simulink library "inp"  (R2021b)
settings: Solver=VariableStepAuto  StartTime=0.0  StopTime=10.0  RelTol=1e-3
undefined symbols (not defined in the file): C_TASK_5MS_S, FALSE, KINP_AcoreReadyToSlp_flg_ovrdflg, KINP_AcoreReadyToSlp_flg_ovrdval, KINP_AllowMovThd_OTA_enum_ovrdflg, KINP_AllowMovThd_OTA_enum_ovrdval, KINP_APSAngleTarget_Deg_ovrdflg, KINP_APSAngleTarget_Deg_ovrdval, KINP_APSDecReq_mps2_ovrdflg, KINP_APSDecReq_mps2_ovrdval, KINP_APSDecReqA_flg_ovrdflg, KINP_APSDecReqA_flg_ovrdval, KINP_APSDFLL_cm_ovrdflg, KINP_APSDFLL_cm_ovrdval, KINP_APSDFLR_cm_ovrdflg, KINP_APSDFLR_cm_ovrdval, KINP_APSDRLL_cm_ovrdflg, KINP_APSDRLL_cm_ovrdval, KINP_APSDRLR_cm_ovrdflg, KINP_APSDRLR_cm_ovrdval, KINP_APSExitCondition_enum_ovrdflg, KINP_APSExitCondition_enum_ovrdval, KINP_APSHWVer_enum_ovrdflg, KINP_APSHWVer_enum_ovrdval, KINP_APSProgressPCT_pct_ovrdflg, KINP_APSProgressPCT_pct_ovrdval, KINP_APSPwrReq_enum_ovrdflg, KINP_APSPwrReq_enum_ovrdval, KINP_APSReq_enum_ovrdflg, KINP_APSReq_enum_ovrdval, KINP_APSRQDisplay_enum_ovrdflg, KINP_APSRQDisplay_enum_ovrdval, KINP_APSRqEPASCtrl_flg_ovrdflg, KINP_APSRqEPASCtrl_flg_ovrdval, KINP_APSShiftPosnReq_enum_ovrdval, KINP_APSShiftPosnReq_enum_ovrflg, KINP_APSSpeedCMD_kph_ovrdval, KINP_APSSpeedCMD_kph_ovrflg, KINP_APSStaSystem_enum_ovrdflg, KINP_APSStaSystem_enum_ovrdval, KINP_APSSWVer_enum_ovrdflg, KINP_APSSWVer_enum_ovrdval, KINP_APSVMCReqA_flg_ovrdval, KINP_APSVMCReqA_flg_ovrflg, KINP_APSVRqEPASCtrl_flg_ovrdflg, KINP_APSVRqEPASCtrl_flg_ovrdval, KINP_AuxBattVolmV_mV_ovrdflg, KINP_AuxBattVolmV_mV_ovrdval, KINP_BTConnectSta_enum_ovrdflg, KINP_BTConnectSta_enum_ovrdval, KINP_CAASSta_enum_ovrdflg, KINP_CAASSta_enum_ovrdval, KINP_CAASVMCReqA_flg_ovrdval, KINP_CAASVMCReqA_flg_ovrflg, KINP_CAN1BusOff_flg_ovrdflg, KINP_CAN1BusOff_flg_ovrdval, KINP_CAN2BusOff_flg_ovrdflg, KINP_CAN2BusOff_flg_ovrdval, KINP_CAN3BusOff_flg_ovrdflg, KINP_CAN3BusOff_flg_ovrdval ... (+222)
libraries: FVT_lib x1035, hcu_lib x1
(part 25 of 33)

== system inp/INP/CAN3/SignalCheck/MCU_N_R2 ==
  BHAL_outputs : Inport
  inp_CanValid_bus : Inport  Port=2
  RrCoolanttempReqNidec : FVT_lib/inp/can_signal_template  SystemSampleTime=-1  VariantActivationTime=update diagram  Latency=0  AutoFrameSizeCalculation=off
      link override defval: Value=KINP_RrCoolanttempReqNidec_cnt_defval
      link override ovrdflg: Value=KINP_RrCoolanttempReqNidec_cnt_ovrdflg
      link override ovrdval: Value=KINP_RrCoolanttempReqNidec_cnt_ovrdval
  RrEOPSpdSetNidec : FVT_lib/inp/can_signal_template  SystemSampleTime=-1  VariantActivationTime=update diagram  Latency=0  AutoFrameSizeCalculation=off
      link override defval: Value=KINP_RrEOPSpdSetNidec_rpm_defval
      link override ovrdflg: Value=KINP_RrEOPSpdSetNidec_rpm_ovrdflg
      link override ovrdval: Value=KINP_RrEOPSpdSetNidec_rpm_ovrdval
  RrFailcode1Nidec : FVT_lib/inp/can_signal_template  SystemSampleTime=-1  VariantActivationTime=update diagram  Latency=0  AutoFrameSizeCalculation=off
      link override defval: Value=KINP_RrFailcode1Nidec_enum_defval
      link override ovrdflg: Value=KINP_RrFailcode1Nidec_enum_ovrdflg
      link override ovrdval: Value=KINP_RrFailcode1Nidec_enum_ovrdval
  RrFailcode2Nidec : FVT_lib/inp/can_signal_template  SystemSampleTime=-1  VariantActivationTime=update diagram  Latency=0  AutoFrameSizeCalculation=off
      link override defval: Value=KINP_RrFailcode2Nidec_enum_defval
      link override ovrdflg: Value=KINP_RrFailcode2Nidec_enum_ovrdflg
      link override ovrdval: Value=KINP_RrFailcode2Nidec_enum_ovrdval
  RrFailcodehistory1Nidec : FVT_lib/inp/can_signal_template  SystemSampleTime=-1  VariantActivationTime=update diagram  Latency=0  AutoFrameSizeCalculation=off
      link override defval: Value=KINP_RrFailcodehistory1Nidec_enum_defval
      link override ovrdflg: Value=KINP_RrFailcodehistory1Nidec_enum_ovrdflg
      link override ovrdval: Value=KINP_RrFailcodehistory1Nidec_enum_ovrdval
  RrFailcodehistory2Nidec : FVT_lib/inp/can_signal_template  SystemSampleTime=-1  VariantActivationTime=update diagram  Latency=0  AutoFrameSizeCalculation=off
      link override defval: Value=KINP_RrFailcodehistory2Nidec_enum_defval
      link override ovrdflg: Value=KINP_RrFailcodehistory2Nidec_enum_ovrdflg
      link override ovrdval: Value=KINP_RrFailcodehistory2Nidec_enum_ovrdval
  RrLLCTempNidec : FVT_lib/inp/can_signal_template  SystemSampleTime=-1  VariantActivationTime=update diagram  Latency=0  AutoFrameSizeCalculation=off
      link override defval: Value=KINP_RrLLCTempNidec_C_defval
      link override ovrdflg: Value=KINP_RrLLCTempNidec_C_ovrdflg
      link override ovrdval: Value=KINP_RrLLCTempNidec_C_ovrdval
  RrLLCflowReqNidec : FVT_lib/inp/can_signal_template  SystemSampleTime=-1  VariantActivationTime=update diagram  Latency=0  AutoFrameSizeCalculation=off
      link override defval: Value=KINP_RrLLCflowReqNidec_Lpmin_defval
      link override ovrdflg: Value=KINP_RrLLCflowReqNidec_Lpmin_ovrdflg
      link override ovrdval: Value=KINP_RrLLCflowReqNidec_Lpmin_ovrdval
  RrMCUTempWarnNidec : FVT_lib/inp/can_signal_template  SystemSampleTime=-1  VariantActivationTime=update diagram  Latency=0  AutoFrameSizeCalculation=off
      link override defval: Value=KINP_RrMCUTempWarnNidec_enum_defval
      link override ovrdflg: Value=KINP_RrMCUTempWarnNidec_enum_ovrdflg
      link override ovrdval: Value=KINP_RrMCUTempWarnNidec_enum_ovrdval
  RrTMTempWarnNidec : FVT_lib/inp/can_signal_template  SystemSampleTime=-1  VariantActivationTime=update diagram  Latency=0  AutoFrameSizeCalculation=off
      link override defval: Value=KINP_RrTMTempWarnNidec_enum_defval
      link override ovrdflg: Value=KINP_RrTMTempWarnNidec_enum_ovrdflg
      link override ovrdval: Value=KINP_RrTMTempWarnNidec_enum_ovrdval
  Terminator_{1..10} (10 alike) : Terminator
  True_VHAL_RrCoolanttempReqNidec_cnt : Constant  Value=TRUE  OutDataTypeStr=boolean
  True_VHAL_RrEOPSpdSetNidec_rpm : Constant  Value=TRUE  OutDataTypeStr=boolean
  True_VHAL_RrFailcode1Nidec_enum : Constant  Value=TRUE  OutDataTypeStr=boolean
  True_VHAL_RrFailcode2Nidec_enum : Constant  Value=TRUE  OutDataTypeStr=boolean
  True_VHAL_RrFailcodehistory1Nidec_enum : Constant  Value=TRUE  OutDataTypeStr=boolean
  True_VHAL_RrFailcodehistory2Nidec_enum : Constant  Value=TRUE  OutDataTypeStr=boolean
  True_VHAL_RrLLCTempNidec_C : Constant  Value=TRUE  OutDataTypeStr=boolean
  True_VHAL_RrLLCflowReqNidec_Lpmin : Constant  Value=TRUE  OutDataTypeStr=boolean
  True_VHAL_RrMCUTempWarnNidec_enum : Constant  Value=TRUE  OutDataTypeStr=boolean
  True_VHAL_RrTMTempWarnNidec_enum : Constant  Value=TRUE  OutDataTypeStr=boolean
  slr1_{1..10} (10 alike) : BusSelector  OutputSignals=VINP_CANMsgValidMCUNR2_flg
  slr_VHAL_RrCoolanttempReqNidec_cnt : BusSelector  OutputSignals=VHAL_RrCoolanttempReqNidec_cnt
  slr_VHAL_RrEOPSpdSetNidec_rpm : BusSelector  OutputSignals=VHAL_RrEOPSpdSetNidec_rpm
  slr_VHAL_RrFailcode1Nidec_enum : BusSelector  OutputSignals=VHAL_RrFailcode1Nidec_enum
  slr_VHAL_RrFailcode2Nidec_enum : BusSelector  OutputSignals=VHAL_RrFailcode2Nidec_enum
  slr_VHAL_RrFailcodehistory1Nidec_enum : BusSelector  OutputSignals=VHAL_RrFailcodehistory1Nidec_enum
  slr_VHAL_RrFailcodehistory2Nidec_enum : BusSelector  OutputSignals=VHAL_RrFailcodehistory2Nidec_enum
  slr_VHAL_RrLLCTempNidec_C : BusSelector  OutputSignals=VHAL_RrLLCTempNidec_C
  slr_VHAL_RrLLCflowReqNidec_Lpmin : BusSelector  OutputSignals=VHAL_RrLLCflowReqNidec_Lpmin
  slr_VHAL_RrMCUTempWarnNidec_enum : BusSelector  OutputSignals=VHAL_RrMCUTempWarnNidec_enum
  slr_VHAL_RrTMTempWarnNidec_enum : BusSelector  OutputSignals=VHAL_RrTMTempWarnNidec_enum
  VINP_RrCoolanttempReqNidec_cnt : Outport
  VINP_RrEOPSpdSetNidec_rpm : Outport  Port=2
  VINP_RrFailcode1Nidec_enum : Outport  Port=3
  VINP_RrFailcode2Nidec_enum : Outport  Port=4
  VINP_RrFailcodehistory1Nidec_enum : Outport  Port=5
  VINP_RrFailcodehistory2Nidec_enum : Outport  Port=6
  VINP_RrLLCTempNidec_C : Outport  Port=7
  VINP_RrLLCflowReqNidec_Lpmin : Outport  Port=8
  VINP_RrMCUTempWarnNidec_enum : Outport  Port=9
  VINP_RrTMTempWarnNidec_enum : Outport  Port=10
  wires:
  BHAL_outputs/1 -> [BHAL_outputs]
  inp_CanValid_bus/1 -> [inp_CanValid_bus]
  [BHAL_outputs] -> slr_VHAL_RrCoolanttempReqNidec_cnt/1
  slr_VHAL_RrCoolanttempReqNidec_cnt/1 -> RrCoolanttempReqNidec/1  "<VHAL_RrCoolanttempReqNidec_cnt>"
  True_VHAL_RrCoolanttempReqNidec_cnt/1 -> RrCoolanttempReqNidec/2
  [inp_CanValid_bus] -> slr1_1/1
  slr1_1/1 -> RrCoolanttempReqNidec/3  "<VINP_CANMsgValidMCUNR2_flg>"
  RrCoolanttempReqNidec/1 -> VINP_RrCoolanttempReqNidec_cnt/1  "VINP_RrCoolanttempReqNidec_cnt"
  RrCoolanttempReqNidec/2 -> Terminator_1/1
  [BHAL_outputs] -> slr_VHAL_RrEOPSpdSetNidec_rpm/1
  slr_VHAL_RrEOPSpdSetNidec_rpm/1 -> RrEOPSpdSetNidec/1  "<VHAL_RrEOPSpdSetNidec_rpm>"
  True_VHAL_RrEOPSpdSetNidec_rpm/1 -> RrEOPSpdSetNidec/2
  [inp_CanValid_bus] -> slr1_2/1
  slr1_2/1 -> RrEOPSpdSetNidec/3  "<VINP_CANMsgValidMCUNR2_flg>"
  RrEOPSpdSetNidec/1 -> VINP_RrEOPSpdSetNidec_rpm/1  "VINP_RrEOPSpdSetNidec_rpm"
  RrEOPSpdSetNidec/2 -> Terminator_2/1
  [BHAL_outputs] -> slr_VHAL_RrFailcode1Nidec_enum/1
  slr_VHAL_RrFailcode1Nidec_enum/1 -> RrFailcode1Nidec/1  "<VHAL_RrFailcode1Nidec_enum>"
  True_VHAL_RrFailcode1Nidec_enum/1 -> RrFailcode1Nidec/2
  [inp_CanValid_bus] -> slr1_3/1
  slr1_3/1 -> RrFailcode1Nidec/3  "<VINP_CANMsgValidMCUNR2_flg>"
  RrFailcode1Nidec/1 -> VINP_RrFailcode1Nidec_enum/1  "VINP_RrFailcode1Nidec_enum"
  RrFailcode1Nidec/2 -> Terminator_3/1
  [BHAL_outputs] -> slr_VHAL_RrFailcode2Nidec_enum/1
  slr_VHAL_RrFailcode2Nidec_enum/1 -> RrFailcode2Nidec/1  "<VHAL_RrFailcode2Nidec_enum>"
  True_VHAL_RrFailcode2Nidec_enum/1 -> RrFailcode2Nidec/2
  [inp_CanValid_bus] -> slr1_4/1
  slr1_4/1 -> RrFailcode2Nidec/3  "<VINP_CANMsgValidMCUNR2_flg>"
  RrFailcode2Nidec/1 -> VINP_RrFailcode2Nidec_enum/1  "VINP_RrFailcode2Nidec_enum"
  RrFailcode2Nidec/2 -> Terminator_4/1
  [BHAL_outputs] -> slr_VHAL_RrFailcodehistory1Nidec_enum/1
  slr_VHAL_RrFailcodehistory1Nidec_enum/1 -> RrFailcodehistory1Nidec/1  "<VHAL_RrFailcodehistory1Nidec_enum>"
  True_VHAL_RrFailcodehistory1Nidec_enum/1 -> RrFailcodehistory1Nidec/2
  [inp_CanValid_bus] -> slr1_5/1
  slr1_5/1 -> RrFailcodehistory1Nidec/3  "<VINP_CANMsgValidMCUNR2_flg>"
  RrFailcodehistory1Nidec/1 -> VINP_RrFailcodehistory1Nidec_enum/1  "VINP_RrFailcodehistory1Nidec_enum"
  RrFailcodehistory1Nidec/2 -> Terminator_5/1
  [BHAL_outputs] -> slr_VHAL_RrFailcodehistory2Nidec_enum/1
  slr_VHAL_RrFailcodehistory2Nidec_enum/1 -> RrFailcodehistory2Nidec/1  "<VHAL_RrFailcodehistory2Nidec_enum>"
  True_VHAL_RrFailcodehistory2Nidec_enum/1 -> RrFailcodehistory2Nidec/2
  [inp_CanValid_bus] -> slr1_6/1
  slr1_6/1 -> RrFailcodehistory2Nidec/3  "<VINP_CANMsgValidMCUNR2_flg>"
  RrFailcodehistory2Nidec/1 -> VINP_RrFailcodehistory2Nidec_enum/1  "VINP_RrFailcodehistory2Nidec_enum"
  RrFailcodehistory2Nidec/2 -> Terminator_6/1
  [BHAL_outputs] -> slr_VHAL_RrLLCTempNidec_C/1
  slr_VHAL_RrLLCTempNidec_C/1 -> RrLLCTempNidec/1  "<VHAL_RrLLCTempNidec_C>"
  True_VHAL_RrLLCTempNidec_C/1 -> RrLLCTempNidec/2
  [inp_CanValid_bus] -> slr1_7/1
  slr1_7/1 -> RrLLCTempNidec/3  "<VINP_CANMsgValidMCUNR2_flg>"
  RrLLCTempNidec/1 -> VINP_RrLLCTempNidec_C/1  "VINP_RrLLCTempNidec_C"
  RrLLCTempNidec/2 -> Terminator_7/1
  [BHAL_outputs] -> slr_VHAL_RrLLCflowReqNidec_Lpmin/1
  slr_VHAL_RrLLCflowReqNidec_Lpmin/1 -> RrLLCflowReqNidec/1  "<VHAL_RrLLCflowReqNidec_Lpmin>"
  True_VHAL_RrLLCflowReqNidec_Lpmin/1 -> RrLLCflowReqNidec/2
  [inp_CanValid_bus] -> slr1_8/1
  slr1_8/1 -> RrLLCflowReqNidec/3  "<VINP_CANMsgValidMCUNR2_flg>"
  RrLLCflowReqNidec/1 -> VINP_RrLLCflowReqNidec_Lpmin/1  "VINP_RrLLCflowReqNidec_Lpmin"
  RrLLCflowReqNidec/2 -> Terminator_8/1
  [BHAL_outputs] -> slr_VHAL_RrMCUTempWarnNidec_enum/1
  slr_VHAL_RrMCUTempWarnNidec_enum/1 -> RrMCUTempWarnNidec/1  "<VHAL_RrMCUTempWarnNidec_enum>"
  True_VHAL_RrMCUTempWarnNidec_enum/1 -> RrMCUTempWarnNidec/2
  [inp_CanValid_bus] -> slr1_9/1
  slr1_9/1 -> RrMCUTempWarnNidec/3  "<VINP_CANMsgValidMCUNR2_flg>"
  RrMCUTempWarnNidec/1 -> VINP_RrMCUTempWarnNidec_enum/1  "VINP_RrMCUTempWarnNidec_enum"
  RrMCUTempWarnNidec/2 -> Terminator_9/1
  [BHAL_outputs] -> slr_VHAL_RrTMTempWarnNidec_enum/1
  slr_VHAL_RrTMTempWarnNidec_enum/1 -> RrTMTempWarnNidec/1  "<VHAL_RrTMTempWarnNidec_enum>"
  True_VHAL_RrTMTempWarnNidec_enum/1 -> RrTMTempWarnNidec/2
  [inp_CanValid_bus] -> slr1_10/1
  slr1_10/1 -> RrTMTempWarnNidec/3  "<VINP_CANMsgValidMCUNR2_flg>"
  RrTMTempWarnNidec/1 -> VINP_RrTMTempWarnNidec_enum/1  "VINP_RrTMTempWarnNidec_enum"
  RrTMTempWarnNidec/2 -> Terminator_10/1

== system inp/INP/CAN3/SignalCheck/MCU_N_R3 ==
  BHAL_outputs : Inport
  inp_CanValid_bus : Inport  Port=2
  RrMCU3HWVerNidec : FVT_lib/inp/can_signal_template  SystemSampleTime=-1  VariantActivationTime=update diagram  Latency=0  AutoFrameSizeCalculation=off
      link override defval: Value=KINP_RrMCU3HWVerNidec_enum_defval
      link override ovrdflg: Value=KINP_RrMCU3HWVerNidec_enum_ovrdflg
      link override ovrdval: Value=KINP_RrMCU3HWVerNidec_enum_ovrdval
  RrMCU3SWVerNidec : FVT_lib/inp/can_signal_template  SystemSampleTime=-1  VariantActivationTime=update diagram  Latency=0  AutoFrameSizeCalculation=off
      link override defval: Value=KINP_RrMCU3SWVerNidec_enum_defval
      link override ovrdflg: Value=KINP_RrMCU3SWVerNidec_enum_ovrdflg
      link override ovrdval: Value=KINP_RrMCU3SWVerNidec_enum_ovrdval
  Terminator_1 : Terminator
  Terminator_2 : Terminator
  True_VHAL_RrMCU3HWVerNidec_enum : Constant  Value=TRUE  OutDataTypeStr=boolean
  True_VHAL_RrMCU3SWVerNidec_enum : Constant  Value=TRUE  OutDataTypeStr=boolean
  slr1_1 : BusSelector  OutputSignals=VINP_CANMsgValidMCUNR3_flg
  slr1_2 : BusSelector  OutputSignals=VINP_CANMsgValidMCUNR3_flg
  slr_VHAL_RrMCU3HWVerNidec_enum : BusSelector  OutputSignals=VHAL_RrMCU3HWVerNidec_enum
  slr_VHAL_RrMCU3SWVerNidec_enum : BusSelector  OutputSignals=VHAL_RrMCU3SWVerNidec_enum
  VINP_RrMCU3HWVerNidec_enum : Outport
  VINP_RrMCU3SWVerNidec_enum : Outport  Port=2
  wires:
  BHAL_outputs/1 -> [BHAL_outputs]
  inp_CanValid_bus/1 -> [inp_CanValid_bus]
  [BHAL_outputs] -> slr_VHAL_RrMCU3HWVerNidec_enum/1
  slr_VHAL_RrMCU3HWVerNidec_enum/1 -> RrMCU3HWVerNidec/1  "<VHAL_RrMCU3HWVerNidec_enum>"
  True_VHAL_RrMCU3HWVerNidec_enum/1 -> RrMCU3HWVerNidec/2
  [inp_CanValid_bus] -> slr1_1/1
  slr1_1/1 -> RrMCU3HWVerNidec/3  "<VINP_CANMsgValidMCUNR3_flg>"
  RrMCU3HWVerNidec/1 -> VINP_RrMCU3HWVerNidec_enum/1  "VINP_RrMCU3HWVerNidec_enum"
  RrMCU3HWVerNidec/2 -> Terminator_1/1
  [BHAL_outputs] -> slr_VHAL_RrMCU3SWVerNidec_enum/1
  slr_VHAL_RrMCU3SWVerNidec_enum/1 -> RrMCU3SWVerNidec/1  "<VHAL_RrMCU3SWVerNidec_enum>"
  True_VHAL_RrMCU3SWVerNidec_enum/1 -> RrMCU3SWVerNidec/2
  [inp_CanValid_bus] -> slr1_2/1
  slr1_2/1 -> RrMCU3SWVerNidec/3  "<VINP_CANMsgValidMCUNR3_flg>"
  RrMCU3SWVerNidec/1 -> VINP_RrMCU3SWVerNidec_enum/1  "VINP_RrMCU3SWVerNidec_enum"
  RrMCU3SWVerNidec/2 -> Terminator_2/1

== system inp/INP/CAN3/SignalCheck/Shifter1 ==
  BHAL_outputs : Inport
  inp_CanValid_bus : Inport  Port=2
  Shifter1CSErr : FVT_lib/inp/can_signal_template  SystemSampleTime=-1  VariantActivationTime=update diagram  Latency=0  AutoFrameSizeCalculation=off
      link override defval: Value=KINP_Shifter1CSErr_flg_defval
      link override ovrdflg: Value=KINP_Shifter1CSErr_flg_ovrdflg
      link override ovrdval: Value=KINP_Shifter1CSErr_flg_ovrdval
  Shifter1RCErr : FVT_lib/inp/can_signal_template  SystemSampleTime=-1  VariantActivationTime=update diagram  Latency=0  AutoFrameSizeCalculation=off
      link override defval: Value=KINP_Shifter1RCErr_flg_defval
      link override ovrdflg: Value=KINP_Shifter1RCErr_flg_ovrdflg
      link override ovrdval: Value=KINP_Shifter1RCErr_flg_ovrdval
  ShifterCRC8 : FVT_lib/inp/can_signal_template  SystemSampleTime=-1  VariantActivationTime=update diagram  Latency=0  AutoFrameSizeCalculation=off
      link override defval: Value=KINP_ShifterCRC8_enum_defval
      link override ovrdflg: Value=KINP_ShifterCRC8_enum_ovrdflg
      link override ovrdval: Value=KINP_ShifterCRC8_enum_ovrdval
  ShifterFailsta : FVT_lib/inp/can_signal_template  SystemSampleTime=-1  VariantActivationTime=update diagram  Latency=0  AutoFrameSizeCalculation=off
      link override defval: Value=KINP_ShifterFailsta_enum_defval
      link override ovrdflg: Value=KINP_ShifterFailsta_enum_ovrdflg
      link override ovrdval: Value=KINP_ShifterFailsta_enum_ovrdval
  ShifterHandleCmd : FVT_lib/inp/can_signal_template  SystemSampleTime=-1  VariantActivationTime=update diagram  Latency=0  AutoFrameSizeCalculation=off
      link override defval: Value=KINP_ShifterHandleCmd_enum_defval
      link override ovrdflg: Value=KINP_ShifterHandleCmd_enum_ovrdflg
      link override ovrdval: Value=KINP_ShifterHandleCmd_enum_ovrdval
  ShifterRC : FVT_lib/inp/can_signal_template  SystemSampleTime=-1  VariantActivationTime=update diagram  Latency=0  AutoFrameSizeCalculation=off
      link override defval: Value=KINP_ShifterRC_enum_defval
      link override ovrdflg: Value=KINP_ShifterRC_enum_ovrdflg
      link override ovrdval: Value=KINP_ShifterRC_enum_ovrdval
  Terminator_{1..6} (6 alike) : Terminator
  True_VHAL_Shifter1CSErr_flg : Constant  Value=TRUE  OutDataTypeStr=boolean
  True_VHAL_Shifter1RCErr_flg : Constant  Value=TRUE  OutDataTypeStr=boolean
  True_VHAL_ShifterCRC8_enum : Constant  Value=TRUE  OutDataTypeStr=boolean
  True_VHAL_ShifterFailsta_enum : Constant  Value=TRUE  OutDataTypeStr=boolean
  True_VHAL_ShifterHandleCmd_enum : Constant  Value=TRUE  OutDataTypeStr=boolean
  True_VHAL_ShifterRC_enum : Constant  Value=TRUE  OutDataTypeStr=boolean
  slr1_{1..6} (6 alike) : BusSelector  OutputSignals=VINP_CANMsgValidShifter1_flg
  slr_VHAL_Shifter1CSErr_flg : BusSelector  OutputSignals=VHAL_Shifter1CSErr_flg
  slr_VHAL_Shifter1RCErr_flg : BusSelector  OutputSignals=VHAL_Shifter1RCErr_flg
  slr_VHAL_ShifterCRC8_enum : BusSelector  OutputSignals=VHAL_ShifterCRC8_enum
  slr_VHAL_ShifterFailsta_enum : BusSelector  OutputSignals=VHAL_ShifterFailsta_enum
  slr_VHAL_ShifterHandleCmd_enum : BusSelector  OutputSignals=VHAL_ShifterHandleCmd_enum
  slr_VHAL_ShifterRC_enum : BusSelector  OutputSignals=VHAL_ShifterRC_enum
  VINP_Shifter1CSErr_flg : Outport
  VINP_Shifter1RCErr_flg : Outport  Port=2
  VINP_ShifterCRC8_enum : Outport  Port=3
  VINP_ShifterFailsta_enum : Outport  Port=4
  VINP_ShifterHandleCmd_enum : Outport  Port=5
  VINP_ShifterRC_enum : Outport  Port=6
  wires:
  BHAL_outputs/1 -> [BHAL_outputs]
  inp_CanValid_bus/1 -> [inp_CanValid_bus]
  [BHAL_outputs] -> slr_VHAL_Shifter1CSErr_flg/1
  slr_VHAL_Shifter1CSErr_flg/1 -> Shifter1CSErr/1  "<VHAL_Shifter1CSErr_flg>"
  True_VHAL_Shifter1CSErr_flg/1 -> Shifter1CSErr/2
  [inp_CanValid_bus] -> slr1_1/1
  slr1_1/1 -> Shifter1CSErr/3  "<VINP_CANMsgValidShifter1_flg>"
  Shifter1CSErr/1 -> VINP_Shifter1CSErr_flg/1  "VINP_Shifter1CSErr_flg"
  Shifter1CSErr/2 -> Terminator_1/1
  [BHAL_outputs] -> slr_VHAL_Shifter1RCErr_flg/1
  slr_VHAL_Shifter1RCErr_flg/1 -> Shifter1RCErr/1  "<VHAL_Shifter1RCErr_flg>"
  True_VHAL_Shifter1RCErr_flg/1 -> Shifter1RCErr/2
  [inp_CanValid_bus] -> slr1_2/1
  slr1_2/1 -> Shifter1RCErr/3  "<VINP_CANMsgValidShifter1_flg>"
  Shifter1RCErr/1 -> VINP_Shifter1RCErr_flg/1  "VINP_Shifter1RCErr_flg"
  Shifter1RCErr/2 -> Terminator_2/1
  [BHAL_outputs] -> slr_VHAL_ShifterCRC8_enum/1
  slr_VHAL_ShifterCRC8_enum/1 -> ShifterCRC8/1  "<VHAL_ShifterCRC8_enum>"
  True_VHAL_ShifterCRC8_enum/1 -> ShifterCRC8/2
  [inp_CanValid_bus] -> slr1_3/1
  slr1_3/1 -> ShifterCRC8/3  "<VINP_CANMsgValidShifter1_flg>"
  ShifterCRC8/1 -> VINP_ShifterCRC8_enum/1  "VINP_ShifterCRC8_enum"
  ShifterCRC8/2 -> Terminator_3/1
  [BHAL_outputs] -> slr_VHAL_ShifterFailsta_enum/1
  slr_VHAL_ShifterFailsta_enum/1 -> ShifterFailsta/1  "<VHAL_ShifterFailsta_enum>"
  True_VHAL_ShifterFailsta_enum/1 -> ShifterFailsta/2
  [inp_CanValid_bus] -> slr1_4/1
  slr1_4/1 -> ShifterFailsta/3  "<VINP_CANMsgValidShifter1_flg>"
  ShifterFailsta/1 -> VINP_ShifterFailsta_enum/1  "VINP_ShifterFailsta_enum"
  ShifterFailsta/2 -> Terminator_4/1
  [BHAL_outputs] -> slr_VHAL_ShifterHandleCmd_enum/1
  slr_VHAL_ShifterHandleCmd_enum/1 -> ShifterHandleCmd/1  "<VHAL_ShifterHandleCmd_enum>"
  True_VHAL_ShifterHandleCmd_enum/1 -> ShifterHandleCmd/2
  [inp_CanValid_bus] -> slr1_5/1
  slr1_5/1 -> ShifterHandleCmd/3  "<VINP_CANMsgValidShifter1_flg>"
  ShifterHandleCmd/1 -> VINP_ShifterHandleCmd_enum/1  "VINP_ShifterHandleCmd_enum"
  ShifterHandleCmd/2 -> Terminator_5/1
  [BHAL_outputs] -> slr_VHAL_ShifterRC_enum/1
  slr_VHAL_ShifterRC_enum/1 -> ShifterRC/1  "<VHAL_ShifterRC_enum>"
  True_VHAL_ShifterRC_enum/1 -> ShifterRC/2
  [inp_CanValid_bus] -> slr1_6/1
  slr1_6/1 -> ShifterRC/3  "<VINP_CANMsgValidShifter1_flg>"
  ShifterRC/1 -> VINP_ShifterRC_enum/1  "VINP_ShifterRC_enum"
  ShifterRC/2 -> Terminator_6/1

== system inp/INP/CAN3/SignalCheck/Shifter2 ==
  BHAL_outputs : Inport
  inp_CanValid_bus : Inport  Port=2
  CSW2DimSwSta : FVT_lib/inp/can_signal_template  SystemSampleTime=-1  VariantActivationTime=update diagram  Latency=0  AutoFrameSizeCalculation=off
      link override defval: Value=KINP_CSW2DimSwSta_flg_defval
      link override ovrdflg: Value=KINP_CSW2DimSwSta_flg_ovrdflg
      link override ovrdval: Value=KINP_CSW2DimSwSta_flg_ovrdval
  CSW2FWasSwSta : FVT_lib/inp/can_signal_template  SystemSampleTime=-1  VariantActivationTime=update diagram  Latency=0  AutoFrameSizeCalculation=off
      link override defval: Value=KINP_CSW2FWasSwSta_enum_defval
      link override ovrdflg: Value=KINP_CSW2FWasSwSta_enum_ovrdflg
      link override ovrdval: Value=KINP_CSW2FWasSwSta_enum_ovrdval
  CSW2FWipSwSta : FVT_lib/inp/can_signal_template  SystemSampleTime=-1  VariantActivationTime=update diagram  Latency=0  AutoFrameSizeCalculation=off
      link override defval: Value=KINP_CSW2FWipSwSta_enum_defval
      link override ovrdflg: Value=KINP_CSW2FWipSwSta_enum_ovrdflg
      link override ovrdval: Value=KINP_CSW2FWipSwSta_enum_ovrdval
  CSW2PassSWSta : FVT_lib/inp/can_signal_template  SystemSampleTime=-1  VariantActivationTime=update diagram  Latency=0  AutoFrameSizeCalculation=off
      link override defval: Value=KINP_CSW2PassSWSta_flg_defval
      link override ovrdflg: Value=KINP_CSW2PassSWSta_flg_ovrdflg
      link override ovrdval: Value=KINP_CSW2PassSWSta_flg_ovrdval
  CSW2RWipWasSwSta : FVT_lib/inp/can_signal_template  SystemSampleTime=-1  VariantActivationTime=update diagram  Latency=0  AutoFrameSizeCalculation=off
      link override defval: Value=KINP_CSW2RWipWasSwSta_enum_defval
      link override ovrdflg: Value=KINP_CSW2RWipWasSwSta_enum_ovrdflg
      link override ovrdval: Value=KINP_CSW2RWipWasSwSta_enum_ovrdval
  CSW2TurnSwSta : FVT_lib/inp/can_signal_template  SystemSampleTime=-1  VariantActivationTime=update diagram  Latency=0  AutoFrameSizeCalculation=off
      link override defval: Value=KINP_CSW2TurnSwSta_enum_defval
      link override ovrdflg: Value=KINP_CSW2TurnSwSta_enum_ovrdflg
      link override ovrdval: Value=KINP_CSW2TurnSwSta_enum_ovrdval
  Shifter2CSErr : FVT_lib/inp/can_signal_template  SystemSampleTime=-1  VariantActivationTime=update diagram  Latency=0  AutoFrameSizeCalculation=off
      link override defval: Value=KINP_Shifter2CSErr_flg_defval
      link override ovrdflg: Value=KINP_Shifter2CSErr_flg_ovrdflg
      link override ovrdval: Value=KINP_Shifter2CSErr_flg_ovrdval
  Shifter2RCErr : FVT_lib/inp/can_signal_template  SystemSampleTime=-1  VariantActivationTime=update diagram  Latency=0  AutoFrameSizeCalculation=off
      link override defval: Value=KINP_Shifter2RCErr_flg_defval
      link override ovrdflg: Value=KINP_Shifter2RCErr_flg_ovrdflg
      link override ovrdval: Value=KINP_Shifter2RCErr_flg_ovrdval
  Terminator_{1..8} (8 alike) : Terminator
  True_VHAL_CSW2DimSwSta_flg : Constant  Value=TRUE  OutDataTypeStr=boolean
  True_VHAL_CSW2FWasSwSta_enum : Constant  Value=TRUE  OutDataTypeStr=boolean
  True_VHAL_CSW2FWipSwSta_enum : Constant  Value=TRUE  OutDataTypeStr=boolean
  True_VHAL_CSW2PassSWSta_flg : Constant  Value=TRUE  OutDataTypeStr=boolean
  True_VHAL_CSW2RWipWasSwSta_enum : Constant  Value=TRUE  OutDataTypeStr=boolean
  True_VHAL_CSW2TurnSwSta_enum : Constant  Value=TRUE  OutDataTypeStr=boolean
  True_VHAL_Shifter2CSErr_flg : Constant  Value=TRUE  OutDataTypeStr=boolean
  True_VHAL_Shifter2RCErr_flg : Constant  Value=TRUE  OutDataTypeStr=boolean
  slr1_{1..8} (8 alike) : BusSelector  OutputSignals=VINP_CANMsgValidShifter2_flg
  slr_VHAL_CSW2DimSwSta_flg : BusSelector  OutputSignals=VHAL_CSW2DimSwSta_flg
  slr_VHAL_CSW2FWasSwSta_enum : BusSelector  OutputSignals=VHAL_CSW2FWasSwSta_enum
  slr_VHAL_CSW2FWipSwSta_enum : BusSelector  OutputSignals=VHAL_CSW2FWipSwSta_enum
  slr_VHAL_CSW2PassSWSta_flg : BusSelector  OutputSignals=VHAL_CSW2PassSWSta_flg
  slr_VHAL_CSW2RWipWasSwSta_enum : BusSelector  OutputSignals=VHAL_CSW2RWipWasSwSta_enum
  slr_VHAL_CSW2TurnSwSta_enum : BusSelector  OutputSignals=VHAL_CSW2TurnSwSta_enum
  slr_VHAL_Shifter2CSErr_flg : BusSelector  OutputSignals=VHAL_Shifter2CSErr_flg
  slr_VHAL_Shifter2RCErr_flg : BusSelector  OutputSignals=VHAL_Shifter2RCErr_flg
  VINP_Shifter2CSErr_flg : Outport
  VINP_Shifter2RCErr_flg : Outport  Port=2
  VINP_CSW2DimSwSta_flg : Outport  Port=3
  VINP_CSW2FWasSwSta_enum : Outport  Port=4
  VINP_CSW2FWipSwSta_enum : Outport  Port=5
  VINP_CSW2PassSWSta_flg : Outport  Port=6
  VINP_CSW2RWipWasSwSta_enum : Outport  Port=7
  VINP_CSW2TurnSwSta_enum : Outport  Port=8
  wires:
  BHAL_outputs/1 -> [BHAL_outputs]
  inp_CanValid_bus/1 -> [inp_CanValid_bus]
  [BHAL_outputs] -> slr_VHAL_Shifter2CSErr_flg/1
  slr_VHAL_Shifter2CSErr_flg/1 -> Shifter2CSErr/1  "<VHAL_Shifter2CSErr_flg>"
  True_VHAL_Shifter2CSErr_flg/1 -> Shifter2CSErr/2
  [inp_CanValid_bus] -> slr1_1/1
  slr1_1/1 -> Shifter2CSErr/3  "<VINP_CANMsgValidShifter2_flg>"
  Shifter2CSErr/1 -> VINP_Shifter2CSErr_flg/1  "VINP_Shifter2CSErr_flg"
  Shifter2CSErr/2 -> Terminator_1/1
  [BHAL_outputs] -> slr_VHAL_Shifter2RCErr_flg/1
  slr_VHAL_Shifter2RCErr_flg/1 -> Shifter2RCErr/1  "<VHAL_Shifter2RCErr_flg>"
  True_VHAL_Shifter2RCErr_flg/1 -> Shifter2RCErr/2
  [inp_CanValid_bus] -> slr1_2/1
  slr1_2/1 -> Shifter2RCErr/3  "<VINP_CANMsgValidShifter2_flg>"
  Shifter2RCErr/1 -> VINP_Shifter2RCErr_flg/1  "VINP_Shifter2RCErr_flg"
  Shifter2RCErr/2 -> Terminator_2/1
  [BHAL_outputs] -> slr_VHAL_CSW2DimSwSta_flg/1
  slr_VHAL_CSW2DimSwSta_flg/1 -> CSW2DimSwSta/1  "<VHAL_CSW2DimSwSta_flg>"
  True_VHAL_CSW2DimSwSta_flg/1 -> CSW2DimSwSta/2
  [inp_CanValid_bus] -> slr1_3/1
  slr1_3/1 -> CSW2DimSwSta/3  "<VINP_CANMsgValidShifter2_flg>"
  CSW2DimSwSta/1 -> VINP_CSW2DimSwSta_flg/1  "VINP_CSW2DimSwSta_flg"
  CSW2DimSwSta/2 -> Terminator_3/1
  [BHAL_outputs] -> slr_VHAL_CSW2FWasSwSta_enum/1
  slr_VHAL_CSW2FWasSwSta_enum/1 -> CSW2FWasSwSta/1  "<VHAL_CSW2FWasSwSta_enum>"
  True_VHAL_CSW2FWasSwSta_enum/1 -> CSW2FWasSwSta/2
  [inp_CanValid_bus] -> slr1_4/1
  slr1_4/1 -> CSW2FWasSwSta/3  "<VINP_CANMsgValidShifter2_flg>"
  CSW2FWasSwSta/1 -> VINP_CSW2FWasSwSta_enum/1  "VINP_CSW2FWasSwSta_enum"
  CSW2FWasSwSta/2 -> Terminator_4/1
  [BHAL_outputs] -> slr_VHAL_CSW2FWipSwSta_enum/1
  slr_VHAL_CSW2FWipSwSta_enum/1 -> CSW2FWipSwSta/1  "<VHAL_CSW2FWipSwSta_enum>"
  True_VHAL_CSW2FWipSwSta_enum/1 -> CSW2FWipSwSta/2
  [inp_CanValid_bus] -> slr1_5/1
  slr1_5/1 -> CSW2FWipSwSta/3  "<VINP_CANMsgValidShifter2_flg>"
  CSW2FWipSwSta/1 -> VINP_CSW2FWipSwSta_enum/1  "VINP_CSW2FWipSwSta_enum"
  CSW2FWipSwSta/2 -> Terminator_5/1
  [BHAL_outputs] -> slr_VHAL_CSW2PassSWSta_flg/1
  slr_VHAL_CSW2PassSWSta_flg/1 -> CSW2PassSWSta/1  "<VHAL_CSW2PassSWSta_flg>"
  True_VHAL_CSW2PassSWSta_flg/1 -> CSW2PassSWSta/2
  [inp_CanValid_bus] -> slr1_6/1
  slr1_6/1 -> CSW2PassSWSta/3  "<VINP_CANMsgValidShifter2_flg>"
  CSW2PassSWSta/1 -> VINP_CSW2PassSWSta_flg/1  "VINP_CSW2PassSWSta_flg"
  CSW2PassSWSta/2 -> Terminator_6/1
  [BHAL_outputs] -> slr_VHAL_CSW2RWipWasSwSta_enum/1
  slr_VHAL_CSW2RWipWasSwSta_enum/1 -> CSW2RWipWasSwSta/1  "<VHAL_CSW2RWipWasSwSta_enum>"
  True_VHAL_CSW2RWipWasSwSta_enum/1 -> CSW2RWipWasSwSta/2
  [inp_CanValid_bus] -> slr1_7/1
  slr1_7/1 -> CSW2RWipWasSwSta/3  "<VINP_CANMsgValidShifter2_flg>"
  CSW2RWipWasSwSta/1 -> VINP_CSW2RWipWasSwSta_enum/1  "VINP_CSW2RWipWasSwSta_enum"
  CSW2RWipWasSwSta/2 -> Terminator_7/1
  [BHAL_outputs] -> slr_VHAL_CSW2TurnSwSta_enum/1
  slr_VHAL_CSW2TurnSwSta_enum/1 -> CSW2TurnSwSta/1  "<VHAL_CSW2TurnSwSta_enum>"
  True_VHAL_CSW2TurnSwSta_enum/1 -> CSW2TurnSwSta/2
  [inp_CanValid_bus] -> slr1_8/1
  slr1_8/1 -> CSW2TurnSwSta/3  "<VINP_CANMsgValidShifter2_flg>"
  CSW2TurnSwSta/1 -> VINP_CSW2TurnSwSta_enum/1  "VINP_CSW2TurnSwSta_enum"
  CSW2TurnSwSta/2 -> Terminator_8/1

== system inp/INP/CAN4/SignalCheck/BodyZone_DR1 ==
  BHAL_outputs : Inport
  inp_CanValid_bus : Inport  Port=2
  BDDSEATAntiSta : FVT_lib/inp/can_signal_template  SystemSampleTime=-1  VariantActivationTime=update diagram  Latency=0  AutoFrameSizeCalculation=off
      link override defval: Value=KINP_BDDSEATAntiSta_flg_defval
      link override ovrdflg: Value=KINP_BDDSEATAntiSta_flg_ovrdflg
      link override ovrdval: Value=KINP_BDDSEATAntiSta_flg_ovrdval
  BDDSEATEntryFunSta : FVT_lib/inp/can_signal_template  SystemSampleTime=-1  VariantActivationTime=update diagram  Latency=0  AutoFrameSizeCalculation=off
      link override defval: Value=KINP_BDDSEATEntryFunSta_flg_defval
      link override ovrdflg: Value=KINP_BDDSEATEntryFunSta_flg_ovrdflg
      link override ovrdval: Value=KINP_BDDSEATEntryFunSta_flg_ovrdval
  BDDSEATErrorSta : FVT_lib/inp/can_signal_template  SystemSampleTime=-1  VariantActivationTime=update diagram  Latency=0  AutoFrameSizeCalculation=off
      link override defval: Value=KINP_BDDSEATErrorSta_flg_defval
      link override ovrdflg: Value=KINP_BDDSEATErrorSta_flg_ovrdflg
      link override ovrdval: Value=KINP_BDDSEATErrorSta_flg_ovrdval
  BDDSEATMemSetSta : FVT_lib/inp/can_signal_template  SystemSampleTime=-1  VariantActivationTime=update diagram  Latency=0  AutoFrameSizeCalculation=off
      link override defval: Value=KINP_BDDSEATMemSetSta_enum_defval
      link override ovrdflg: Value=KINP_BDDSEATMemSetSta_enum_ovrdflg
      link override ovrdval: Value=KINP_BDDSEATMemSetSta_enum_ovrdval
  BDDSEATModeSta : FVT_lib/inp/can_signal_template  SystemSampleTime=-1  VariantActivationTime=update diagram  Latency=0  AutoFrameSizeCalculation=off
      link override defval: Value=KINP_BDDSEATModeSta_enum_defval
      link override ovrdflg: Value=KINP_BDDSEATModeSta_enum_ovrdflg
      link override ovrdval: Value=KINP_BDDSEATModeSta_enum_ovrdval
  BDDSEATVentSta : FVT_lib/inp/can_signal_template  SystemSampleTime=-1  VariantActivationTime=update diagram  Latency=0  AutoFrameSizeCalculation=off
      link override defval: Value=KINP_BDDSEATVentSta_enum_defval
      link override ovrdflg: Value=KINP_BDDSEATVentSta_enum_ovrdflg
      link override ovrdval: Value=KINP_BDDSEATVentSta_enum_ovrdval
  BDDSEATheaterSta : FVT_lib/inp/can_signal_template  SystemSampleTime=-1  VariantActivationTime=update diagram  Latency=0  AutoFrameSizeCalculation=off
      link override defval: Value=KINP_BDDSEATheaterSta_enum_defval
      link override ovrdflg: Value=KINP_BDDSEATheaterSta_enum_ovrdflg
      link override ovrdval: Value=KINP_BDDSEATheaterSta_enum_ovrdval
  Terminator_{1..7} (7 alike) : Terminator
  True_VHAL_BDDSEATAntiSta_flg : Constant  Value=TRUE  OutDataTypeStr=boolean
  True_VHAL_BDDSEATEntryFunSta_flg : Constant  Value=TRUE  OutDataTypeStr=boolean
  True_VHAL_BDDSEATErrorSta_flg : Constant  Value=TRUE  OutDataTypeStr=boolean
  True_VHAL_BDDSEATMemSetSta_enum : Constant  Value=TRUE  OutDataTypeStr=boolean
  True_VHAL_BDDSEATModeSta_enum : Constant  Value=TRUE  OutDataTypeStr=boolean
  True_VHAL_BDDSEATVentSta_enum : Constant  Value=TRUE  OutDataTypeStr=boolean
  True_VHAL_BDDSEATheaterSta_enum : Constant  Value=TRUE  OutDataTypeStr=boolean
  slr1_{1..7} (7 alike) : BusSelector  OutputSignals=VINP_CANMsgValidBodyZoneDR1_flg
  slr_VHAL_BDDSEATAntiSta_flg : BusSelector  OutputSignals=VHAL_BDDSEATAntiSta_flg
  slr_VHAL_BDDSEATEntryFunSta_flg : BusSelector  OutputSignals=VHAL_BDDSEATEntryFunSta_flg
  slr_VHAL_BDDSEATErrorSta_flg : BusSelector  OutputSignals=VHAL_BDDSEATErrorSta_flg
  slr_VHAL_BDDSEATMemSetSta_enum : BusSelector  OutputSignals=VHAL_BDDSEATMemSetSta_enum
  slr_VHAL_BDDSEATModeSta_enum : BusSelector  OutputSignals=VHAL_BDDSEATModeSta_enum
  slr_VHAL_BDDSEATVentSta_enum : BusSelector  OutputSignals=VHAL_BDDSEATVentSta_enum
  slr_VHAL_BDDSEATheaterSta_enum : BusSelector  OutputSignals=VHAL_BDDSEATheaterSta_enum
  VINP_BDDSEATAntiSta_flg : Outport
  VINP_BDDSEATEntryFunSta_flg : Outport  Port=2
  VINP_BDDSEATErrorSta_flg : Outport  Port=3
  VINP_BDDSEATMemSetSta_enum : Outport  Port=4
  VINP_BDDSEATModeSta_enum : Outport  Port=5
  VINP_BDDSEATVentSta_enum : Outport  Port=6
  VINP_BDDSEATheaterSta_enum : Outport  Port=7
  wires:
  BHAL_outputs/1 -> [BHAL_outputs]
  inp_CanValid_bus/1 -> [inp_CanValid_bus]
  [BHAL_outputs] -> slr_VHAL_BDDSEATAntiSta_flg/1
  slr_VHAL_BDDSEATAntiSta_flg/1 -> BDDSEATAntiSta/1  "<VHAL_BDDSEATAntiSta_flg>"
  True_VHAL_BDDSEATAntiSta_flg/1 -> BDDSEATAntiSta/2
  [inp_CanValid_bus] -> slr1_1/1
  slr1_1/1 -> BDDSEATAntiSta/3  "<VINP_CANMsgValidBodyZoneDR1_flg>"
  BDDSEATAntiSta/1 -> VINP_BDDSEATAntiSta_flg/1  "VINP_BDDSEATAntiSta_flg"
  BDDSEATAntiSta/2 -> Terminator_1/1
  [BHAL_outputs] -> slr_VHAL_BDDSEATEntryFunSta_flg/1
  slr_VHAL_BDDSEATEntryFunSta_flg/1 -> BDDSEATEntryFunSta/1  "<VHAL_BDDSEATEntryFunSta_flg>"
  True_VHAL_BDDSEATEntryFunSta_flg/1 -> BDDSEATEntryFunSta/2
  [inp_CanValid_bus] -> slr1_2/1
  slr1_2/1 -> BDDSEATEntryFunSta/3  "<VINP_CANMsgValidBodyZoneDR1_flg>"
  BDDSEATEntryFunSta/1 -> VINP_BDDSEATEntryFunSta_flg/1  "VINP_BDDSEATEntryFunSta_flg"
  BDDSEATEntryFunSta/2 -> Terminator_2/1
  [BHAL_outputs] -> slr_VHAL_BDDSEATErrorSta_flg/1
  slr_VHAL_BDDSEATErrorSta_flg/1 -> BDDSEATErrorSta/1  "<VHAL_BDDSEATErrorSta_flg>"
  True_VHAL_BDDSEATErrorSta_flg/1 -> BDDSEATErrorSta/2
  [inp_CanValid_bus] -> slr1_3/1
  slr1_3/1 -> BDDSEATErrorSta/3  "<VINP_CANMsgValidBodyZoneDR1_flg>"
  BDDSEATErrorSta/1 -> VINP_BDDSEATErrorSta_flg/1  "VINP_BDDSEATErrorSta_flg"
  BDDSEATErrorSta/2 -> Terminator_3/1
  [BHAL_outputs] -> slr_VHAL_BDDSEATMemSetSta_enum/1
  slr_VHAL_BDDSEATMemSetSta_enum/1 -> BDDSEATMemSetSta/1  "<VHAL_BDDSEATMemSetSta_enum>"
  True_VHAL_BDDSEATMemSetSta_enum/1 -> BDDSEATMemSetSta/2
  [inp_CanValid_bus] -> slr1_4/1
  slr1_4/1 -> BDDSEATMemSetSta/3  "<VINP_CANMsgValidBodyZoneDR1_flg>"
  BDDSEATMemSetSta/1 -> VINP_BDDSEATMemSetSta_enum/1  "VINP_BDDSEATMemSetSta_enum"
  BDDSEATMemSetSta/2 -> Terminator_4/1
  [BHAL_outputs] -> slr_VHAL_BDDSEATModeSta_enum/1
  slr_VHAL_BDDSEATModeSta_enum/1 -> BDDSEATModeSta/1  "<VHAL_BDDSEATModeSta_enum>"
  True_VHAL_BDDSEATModeSta_enum/1 -> BDDSEATModeSta/2
  [inp_CanValid_bus] -> slr1_5/1
  slr1_5/1 -> BDDSEATModeSta/3  "<VINP_CANMsgValidBodyZoneDR1_flg>"
  BDDSEATModeSta/1 -> VINP_BDDSEATModeSta_enum/1  "VINP_BDDSEATModeSta_enum"
  BDDSEATModeSta/2 -> Terminator_5/1
  [BHAL_outputs] -> slr_VHAL_BDDSEATVentSta_enum/1
  slr_VHAL_BDDSEATVentSta_enum/1 -> BDDSEATVentSta/1  "<VHAL_BDDSEATVentSta_enum>"
  True_VHAL_BDDSEATVentSta_enum/1 -> BDDSEATVentSta/2
  [inp_CanValid_bus] -> slr1_6/1
  slr1_6/1 -> BDDSEATVentSta/3  "<VINP_CANMsgValidBodyZoneDR1_flg>"
  BDDSEATVentSta/1 -> VINP_BDDSEATVentSta_enum/1  "VINP_BDDSEATVentSta_enum"
  BDDSEATVentSta/2 -> Terminator_6/1
  [BHAL_outputs] -> slr_VHAL_BDDSEATheaterSta_enum/1
  slr_VHAL_BDDSEATheaterSta_enum/1 -> BDDSEATheaterSta/1  "<VHAL_BDDSEATheaterSta_enum>"
  True_VHAL_BDDSEATheaterSta_enum/1 -> BDDSEATheaterSta/2
  [inp_CanValid_bus] -> slr1_7/1
  slr1_7/1 -> BDDSEATheaterSta/3  "<VINP_CANMsgValidBodyZoneDR1_flg>"
  BDDSEATheaterSta/1 -> VINP_BDDSEATheaterSta_enum/1  "VINP_BDDSEATheaterSta_enum"
  BDDSEATheaterSta/2 -> Terminator_7/1

== system inp/INP/CAN4/SignalCheck/BodyZone_DR2 ==
  BHAL_outputs : Inport
  inp_CanValid_bus : Inport  Port=2
  BDAPMWinFOpenedSta : FVT_lib/inp/can_signal_template  SystemSampleTime=-1  VariantActivationTime=update diagram  Latency=0  AutoFrameSizeCalculation=off
      link override defval: Value=KINP_BDAPMWinFOpenedSta_pct_defval
      link override ovrdflg: Value=KINP_BDAPMWinFOpenedSta_pct_ovrdflg
      link override ovrdval: Value=KINP_BDAPMWinFOpenedSta_pct_ovrdval
  BDAPMWinROpenedSta : FVT_lib/inp/can_signal_template  SystemSampleTime=-1  VariantActivationTime=update diagram  Latency=0  AutoFrameSizeCalculation=off
      link override defval: Value=KINP_BDAPMWinROpenedSta_pct_defval
      link override ovrdflg: Value=KINP_BDAPMWinROpenedSta_pct_ovrdflg
      link override ovrdval: Value=KINP_BDAPMWinROpenedSta_pct_ovrdval
  BDDoorFHandleCloseSta : FVT_lib/inp/can_signal_template  SystemSampleTime=-1  VariantActivationTime=update diagram  Latency=0  AutoFrameSizeCalculation=off
      link override defval: Value=KINP_BDDoorFHandleCloseSta_flg_defval
      link override ovrdflg: Value=KINP_BDDoorFHandleCloseSta_flg_ovrdflg
      link override ovrdval: Value=KINP_BDDoorFHandleCloseSta_flg_ovrdval
  BDDoorRHandleCloseSta : FVT_lib/inp/can_signal_template  SystemSampleTime=-1  VariantActivationTime=update diagram  Latency=0  AutoFrameSizeCalculation=off
      link override defval: Value=KINP_BDDoorRHandleCloseSta_flg_defval
      link override ovrdflg: Value=KINP_BDDoorRHandleCloseSta_flg_ovrdflg
      link override ovrdval: Value=KINP_BDDoorRHandleCloseSta_flg_ovrdval
  Terminator_{1..4} (4 alike) : Terminator
  True_VHAL_BDAPMWinFOpenedSta_pct : Constant  Value=TRUE  OutDataTypeStr=boolean
  True_VHAL_BDAPMWinROpenedSta_pct : Constant  Value=TRUE  OutDataTypeStr=boolean
  True_VHAL_BDDoorFHandleCloseSta_flg : Constant  Value=TRUE  OutDataTypeStr=boolean
  True_VHAL_BDDoorRHandleCloseSta_flg : Constant  Value=TRUE  OutDataTypeStr=boolean
  slr1_{1..4} (4 alike) : BusSelector  OutputSignals=VINP_CANMsgValidBodyZoneDR2_flg
  slr_VHAL_BDAPMWinFOpenedSta_pct : BusSelector  OutputSignals=VHAL_BDAPMWinFOpenedSta_pct
  slr_VHAL_BDAPMWinROpenedSta_pct : BusSelector  OutputSignals=VHAL_BDAPMWinROpenedSta_pct
  slr_VHAL_BDDoorFHandleCloseSta_flg : BusSelector  OutputSignals=VHAL_BDDoorFHandleCloseSta_flg
  slr_VHAL_BDDoorRHandleCloseSta_flg : BusSelector  OutputSignals=VHAL_BDDoorRHandleCloseSta_flg
  VINP_BDAPMWinFOpenedSta_pct : Outport
  VINP_BDAPMWinROpenedSta_pct : Outport  Port=2
  VINP_BDDoorFHandleCloseSta_flg : Outport  Port=3
  VINP_BDDoorRHandleCloseSta_flg : Outport  Port=4
  wires:
  BHAL_outputs/1 -> [BHAL_outputs]
  inp_CanValid_bus/1 -> [inp_CanValid_bus]
  [BHAL_outputs] -> slr_VHAL_BDAPMWinFOpenedSta_pct/1
  slr_VHAL_BDAPMWinFOpenedSta_pct/1 -> BDAPMWinFOpenedSta/1  "<VHAL_BDAPMWinFOpenedSta_pct>"
  True_VHAL_BDAPMWinFOpenedSta_pct/1 -> BDAPMWinFOpenedSta/2
  [inp_CanValid_bus] -> slr1_1/1
  slr1_1/1 -> BDAPMWinFOpenedSta/3  "<VINP_CANMsgValidBodyZoneDR2_flg>"
  BDAPMWinFOpenedSta/1 -> VINP_BDAPMWinFOpenedSta_pct/1  "VINP_BDAPMWinFOpenedSta_pct"
  BDAPMWinFOpenedSta/2 -> Terminator_1/1
  [BHAL_outputs] -> slr_VHAL_BDAPMWinROpenedSta_pct/1
  slr_VHAL_BDAPMWinROpenedSta_pct/1 -> BDAPMWinROpenedSta/1  "<VHAL_BDAPMWinROpenedSta_pct>"
  True_VHAL_BDAPMWinROpenedSta_pct/1 -> BDAPMWinROpenedSta/2
  [inp_CanValid_bus] -> slr1_2/1
  slr1_2/1 -> BDAPMWinROpenedSta/3  "<VINP_CANMsgValidBodyZoneDR2_flg>"
  BDAPMWinROpenedSta/1 -> VINP_BDAPMWinROpenedSta_pct/1  "VINP_BDAPMWinROpenedSta_pct"
  BDAPMWinROpenedSta/2 -> Terminator_2/1
  [BHAL_outputs] -> slr_VHAL_BDDoorFHandleCloseSta_flg/1
  slr_VHAL_BDDoorFHandleCloseSta_flg/1 -> BDDoorFHandleCloseSta/1  "<VHAL_BDDoorFHandleCloseSta_flg>"
  True_VHAL_BDDoorFHandleCloseSta_flg/1 -> BDDoorFHandleCloseSta/2
  [inp_CanValid_bus] -> slr1_3/1
  slr1_3/1 -> BDDoorFHandleCloseSta/3  "<VINP_CANMsgValidBodyZoneDR2_flg>"
  BDDoorFHandleCloseSta/1 -> VINP_BDDoorFHandleCloseSta_flg/1  "VINP_BDDoorFHandleCloseSta_flg"
  BDDoorFHandleCloseSta/2 -> Terminator_3/1
  [BHAL_outputs] -> slr_VHAL_BDDoorRHandleCloseSta_flg/1
  slr_VHAL_BDDoorRHandleCloseSta_flg/1 -> BDDoorRHandleCloseSta/1  "<VHAL_BDDoorRHandleCloseSta_flg>"
  True_VHAL_BDDoorRHandleCloseSta_flg/1 -> BDDoorRHandleCloseSta/2
  [inp_CanValid_bus] -> slr1_4/1
  slr1_4/1 -> BDDoorRHandleCloseSta/3  "<VINP_CANMsgValidBodyZoneDR2_flg>"
  BDDoorRHandleCloseSta/1 -> VINP_BDDoorRHandleCloseSta_flg/1  "VINP_BDDoorRHandleCloseSta_flg"
  BDDoorRHandleCloseSta/2 -> Terminator_4/1
